simulink library "ddm"  (R2021b)
settings: Solver=VariableStepAuto  StartTime=0.0  StopTime=10.0  RelTol=1e-3
undefined symbols (not defined in the file): ADDM_FrTMTqDev_X_Nm, ADDM_RrTMTqDev_X_Nm, ENUM_ADASACCSTA_ERROR, ENUM_ADASACCSTA_OFF, ENUM_ADASACCSTA_STANDBY, ENUM_ALLOWMOV_ALLOWREADY, ENUM_APS, ENUM_BRKSTA_ERROR, ENUM_BRKSTA_OFF, ENUM_BRKSTA_ON, ENUM_BRKSW_INVALID, ENUM_BRKSW_OFF, ENUM_BRKSW_ON, ENUM_CHGPREACTERRSTA_OBCPRE, ENUM_DCDCFAULTSTA_ANYFAULTLV1, ENUM_DCDCFAULTSTA_ANYFAULTLV2, ENUM_DRIVETRAIN_AWD, ENUM_DRIVETRAIN_FWD, ENUM_DRIVETRAIN_RWD, ENUM_EDUDRTSTA_NORMAL, ENUM_EPBERROR_FAILED, ENUM_EPBSTA_APPLIED, ENUM_EPBSTA_RELEASED, ENUM_ESCAPSSta_APSUNAVAILABLE, ENUM_GEARACTUALPOSN_INVALID, ENUM_GEARACTUALPOSN_P, ENUM_HVBATTREADYPRE_READY, ENUM_HWRESETSTA_HWRESETING, ENUM_MCUWARN_LV0, ENUM_MCUWARN_LV1, ENUM_MCUWARN_LV2, ENUM_MCUWARN_LV3, ENUM_MCUWARN_NOERROR, ENUM_OBCFAULTSTA_ANYFAULT, ENUM_PAS_R2F2, ENUM_PDFAULT_BATTPDFAIL, ENUM_PDFAULT_DCDCDISABLE, ENUM_PDFAULT_MCUDISABLE, ENUM_PDFAULT_MCUDISCHRG, ENUM_POWERSTA_OFF, ENUM_POWERSTA_ON, ENUM_POWERSTA_READY, ENUM_POWERSTA_STANDBY, ENUM_PRESSINDI_LOW, ENUM_PUFAULT_BATTUPFAIL, ENUM_PUFAULT_DCDCENABLEFAIL, ENUM_PUFAULT_PRECHRGCHKFAIL, ENUM_PUFAULT_SAFETYCHKFAIL, ENUM_PWRSTASW_OFF, ENUM_PWRSTASW_OFFA, ENUM_PWRSTASW_OFFCHVCHRG, ENUM_PWRSTASW_OFFCLVCHRG, ENUM_PWRSTASW_ON, ENUM_PWRSTASW_ONHVCHRG, ENUM_PWRSTASW_READY, ENUM_PWRSTASW_STANDBY, ENUM_RAPSErrWarnSta_NORMAL, ENUM_RAPSErrWarnSta_RAPSERRLV1, ENUM_SHIFTCOMMAND_P, ENUM_SHIFTERERRSTA_PBUTTONFAILURE ... (+471)
libraries: hcu_lib x540, simulink x3
(part 3 of 26)

== system ddm/DDM/DDM_MCU_Signal_Selector ==
  BINP_CAN3_outputs : Inport  OutDataTypeStr=Bus: BINP_CAN3_outputs
  BINP_SYS_outputs : Inport  Port=2  OutDataTypeStr=Bus: BINP_SYS_outputs
  Bus Creator : BusCreator  Inputs=14
  Bus Selector : BusSelector  OutputSignals=VINP_CANMsgValidMCUBF1_flg,VINP_CANMsgValidMCUNF1_flg,VINP_MCUBF1RCErr_flg,VINP_MCUNF1RCErr_flg,VINP_MCUBF1CSErr_flg,VINP_MCUNF1CSErr_flg,VINP_CANMsgValidMCUBR1_flg,VINP_CANMsgValidMCUNR1_flg,VINP_MCUBR1RCErr_flg,VINP_MCUNR1RCErr_flg,VINP_MCUBR1CSErr_flg,VINP_MCUNR1CSErr_flg,VINP_MCUWarnFNidec_enum,VINP_MCUWarnRNidec_enum,VINP_MCUWarnF_enum,VINP_MCUWarnR_enum,VINP_FrMCUReady4Pre_flg,VINP_FrMCUReady4PreNidec_flg,VINP_RrMCUReady4Pre_flg,VINP_RrMCUReady4PreNidec_flg,VINP_FrMCUEnaSta_flg,VINP_FrMCUEnaStaNidec_flg,VINP_RrMCUEnaSta_flg,VINP_RrMCUEnaStaNidec_flg,VINP_FrMCUDCBusVolt_V,VINP_FrMCUDCBusVoltNidec_V,VINP_RrMCUDCBusVolt_V,VINP_RrMCUDCBusVoltNidec_V
  Bus Selector1 : BusSelector  OutputSignals=VINP_VehicleType_enum
  "DDM Signal Convert " : Subsystem  TreatAsAtomicUnit=on
  BDDM_CAN3MCU_outputs : Outport
  wires:
  BINP_CAN3_outputs/1 -> Bus Selector/1
  [VINP_MCUBF1RCErr_flg] -> "DDM Signal Convert "/3(VINP_MCUBF1RCErr_flg)
  [VINP_RrMCUDCBusVoltNidec_V] -> "DDM Signal Convert "/29(VINP_RrMCUDCBusVoltNidec_V)
  "DDM Signal Convert "/14(VDDM_RrMCUDCBusVolt_V) -> [VDDM_RrMCUDCBusVolt_V]
  [VINP_RrMCUReady4Pre_flg] -> "DDM Signal Convert "/20(VINP_RrMCUReady4Pre_flg)
  "DDM Signal Convert "/4(VDDM_CANMsgValidMCUR1_flg) -> [VDDM_CANMsgValidMCUR1_flg]
  "DDM Signal Convert "/6(VDDM_MCUR1CSErr_flg) -> [VDDM_MCUR1CSErr_flg]
  [VINP_MCUBF1CSErr_flg] -> "DDM Signal Convert "/5(VINP_MCUBF1CSErr_flg)
  [VINP_MCUBR1RCErr_flg] -> "DDM Signal Convert "/9(VINP_MCUBR1RCErr_flg)
  [VINP_MCUBR1CSErr_flg] -> "DDM Signal Convert "/11(VINP_MCUBR1CSErr_flg)
  [VINP_VehicleType_enum] -> "DDM Signal Convert "/13(VINP_VehicleType_enum)
  [VINP_RrMCUDCBusVolt_V] -> "DDM Signal Convert "/28(VINP_RrMCUDCBusVolt_V)
  [VINP_FrMCUEnaStaNidec_flg] -> "DDM Signal Convert "/23(VINP_FrMCUEnaStaNidec_flg)
  [VINP_MCUNR1RCErr_flg] -> "DDM Signal Convert "/10(VINP_MCUNR1RCErr_flg)
  "DDM Signal Convert "/7(VDDM_MCUWarnF_enum) -> [VDDM_MCUWarnF_enum]
  [VINP_MCUWarnR_enum] -> "DDM Signal Convert "/17(VINP_MCUWarnR_enum)
  [VINP_FrMCUReady4PreNidec_flg] -> "DDM Signal Convert "/19(VINP_FrMCUReady4PreNidec_flg)
  [VINP_MCUNR1CSErr_flg] -> "DDM Signal Convert "/12(VINP_MCUNR1CSErr_flg)
  [VINP_RrMCUEnaStaNidec_flg] -> "DDM Signal Convert "/25(VINP_RrMCUEnaStaNidec_flg)
  "DDM Signal Convert "/1(VDDM_CANMsgValidMCUF1_flg) -> [VDDM_CANMsgValidMCUF1_flg]
  [VINP_FrMCUReady4Pre_flg] -> "DDM Signal Convert "/18(VINP_FrMCUReady4Pre_flg)
  [VINP_MCUWarnRNidec_enum] -> "DDM Signal Convert "/15(VINP_MCUWarnRNidec_enum)
  "DDM Signal Convert "/13(VDDM_FrMCUDCBusVolt_V) -> [VDDM_FrMCUDCBusVolt_V]
  [VINP_CANMsgValidMCUNR1_flg] -> "DDM Signal Convert "/8(VINP_CANMsgValidMCUNR1_flg)
  [VINP_FrMCUDCBusVoltNidec_V] -> "DDM Signal Convert "/27(VINP_FrMCUDCBusVoltNidec_V)
  "DDM Signal Convert "/2(VDDM_MCUF1RCErr_flg) -> [VDDM_MCUF1RCErr_flg]
  [VINP_CANMsgValidMCUBR1_flg] -> "DDM Signal Convert "/7(VINP_CANMsgValidMCUBR1_flg)
  [VINP_CANMsgValidMCUNF1_flg] -> "DDM Signal Convert "/2(VINP_CANMsgValidMCUNF1_flg)
  [VINP_CANMsgValidMCUBF1_flg] -> "DDM Signal Convert "/1(VINP_CANMsgValidMCUBF1_flg)
  "DDM Signal Convert "/3(VDDM_MCUF1CSErr_flg) -> [VDDM_MCUF1CSErr_flg]
  [VINP_RrMCUEnaSta_flg] -> "DDM Signal Convert "/24(VINP_RrMCUEnaSta_flg)
  [VINP_MCUNF1RCErr_flg] -> "DDM Signal Convert "/4(VINP_MCUNF1RCErr_flg)
  "DDM Signal Convert "/10(VDDM_RrMCUReady4Pre_flg) -> [VDDM_RrMCUReady4Pre_flg]
  "DDM Signal Convert "/5(VDDM_MCUR1RCErr_flg) -> [VDDM_MCUR1RCErr_flg]
  "DDM Signal Convert "/12(VDDM_RrMCUEnaSta_flg) -> [VDDM_RrMCUEnaSta_flg]
  [VINP_MCUWarnF_enum] -> "DDM Signal Convert "/16(VINP_MCUWarnF_enum)
  "DDM Signal Convert "/9(VDDM_FrMCUReady4Pre_flg) -> [VDDM_FrMCUReady4Pre_flg]
  [VINP_MCUNF1CSErr_flg] -> "DDM Signal Convert "/6(VINP_MCUNF1CSErr_flg)
  "DDM Signal Convert "/8(VDDM_MCUWarnR_enum) -> [VDDM_MCUWarnR_enum]
  [VINP_FrMCUDCBusVolt_V] -> "DDM Signal Convert "/26(VINP_FrMCUDCBusVolt_V)
  [VINP_RrMCUReady4PreNidec_flg] -> "DDM Signal Convert "/21(VINP_RrMCUReady4PreNidec_flg)
  "DDM Signal Convert "/11(VDDM_FrMCUEnaSta_flg) -> [VDDM_FrMCUEnaSta_flg]
  [VINP_FrMCUEnaSta_flg] -> "DDM Signal Convert "/22(VINP_FrMCUEnaSta_flg)
  [VINP_MCUWarnFNidec_enum] -> "DDM Signal Convert "/14(VINP_MCUWarnFNidec_enum)
  Bus Selector/1 -> [VINP_CANMsgValidMCUBF1_flg]  "<VINP_CANMsgValidMCUBF1_flg>"
  Bus Selector/2 -> [VINP_CANMsgValidMCUNF1_flg]  "<VINP_CANMsgValidMCUNF1_flg>"
  Bus Selector/3 -> [VINP_MCUBF1RCErr_flg]  "<VINP_MCUBF1RCErr_flg>"
  Bus Selector/4 -> [VINP_MCUNF1RCErr_flg]  "<VINP_MCUNF1RCErr_flg>"
  Bus Selector/5 -> [VINP_MCUBF1CSErr_flg]  "<VINP_MCUBF1CSErr_flg>"
  Bus Selector/6 -> [VINP_MCUNF1CSErr_flg]  "<VINP_MCUNF1CSErr_flg>"
  Bus Selector/7 -> [VINP_CANMsgValidMCUBR1_flg]  "<VINP_CANMsgValidMCUBR1_flg>"
  Bus Selector/8 -> [VINP_CANMsgValidMCUNR1_flg]  "<VINP_CANMsgValidMCUNR1_flg>"
  Bus Selector/9 -> [VINP_MCUBR1RCErr_flg]  "<VINP_MCUBR1RCErr_flg>"
  Bus Selector/10 -> [VINP_MCUNR1RCErr_flg]  "<VINP_MCUNR1RCErr_flg>"
  Bus Selector/11 -> [VINP_MCUBR1CSErr_flg]  "<VINP_MCUBR1CSErr_flg>"
  Bus Selector/12 -> [VINP_MCUNR1CSErr_flg]  "<VINP_MCUNR1CSErr_flg>"
  Bus Selector/13 -> [VINP_MCUWarnFNidec_enum]  "<VINP_MCUWarnFNidec_enum>"
  Bus Selector/14 -> [VINP_MCUWarnRNidec_enum]  "<VINP_MCUWarnRNidec_enum>"
  Bus Selector/15 -> [VINP_MCUWarnF_enum]  "<VINP_MCUWarnF_enum>"
  Bus Selector/16 -> [VINP_MCUWarnR_enum]  "<VINP_MCUWarnR_enum>"
  Bus Selector/17 -> [VINP_FrMCUReady4Pre_flg]  "<VINP_FrMCUReady4Pre_flg>"
  Bus Selector/18 -> [VINP_FrMCUReady4PreNidec_flg]  "<VINP_FrMCUReady4PreNidec_flg>"
  Bus Selector/19 -> [VINP_RrMCUReady4Pre_flg]  "<VINP_RrMCUReady4Pre_flg>"
  Bus Selector/20 -> [VINP_RrMCUReady4PreNidec_flg]  "<VINP_RrMCUReady4PreNidec_flg>"
  Bus Selector/21 -> [VINP_FrMCUEnaSta_flg]  "<VINP_FrMCUEnaSta_flg>"
  Bus Selector/22 -> [VINP_FrMCUEnaStaNidec_flg]  "<VINP_FrMCUEnaStaNidec_flg>"
  Bus Selector/23 -> [VINP_RrMCUEnaSta_flg]  "<VINP_RrMCUEnaSta_flg>"
  Bus Selector/24 -> [VINP_RrMCUEnaStaNidec_flg]  "<VINP_RrMCUEnaStaNidec_flg>"
  Bus Selector/25 -> [VINP_FrMCUDCBusVolt_V]  "<VINP_FrMCUDCBusVolt_V>"
  Bus Selector/26 -> [VINP_FrMCUDCBusVoltNidec_V]  "<VINP_FrMCUDCBusVoltNidec_V>"
  Bus Selector/27 -> [VINP_RrMCUDCBusVolt_V]  "<VINP_RrMCUDCBusVolt_V>"
  Bus Selector/28 -> [VINP_RrMCUDCBusVoltNidec_V]  "<VINP_RrMCUDCBusVoltNidec_V>"
  BINP_SYS_outputs/1 -> Bus Selector1/1
  Bus Selector1/1 -> [VINP_VehicleType_enum]  "<VINP_VehicleType_enum>"
  Bus Creator/1 -> BDDM_CAN3MCU_outputs/1
  [VDDM_CANMsgValidMCUF1_flg] -> Bus Creator/1
  [VDDM_RrMCUDCBusVolt_V] -> Bus Creator/14
  [VDDM_FrMCUDCBusVolt_V] -> Bus Creator/13
  [VDDM_RrMCUEnaSta_flg] -> Bus Creator/12
  [VDDM_FrMCUEnaSta_flg] -> Bus Creator/11
  [VDDM_RrMCUReady4Pre_flg] -> Bus Creator/10
  [VDDM_FrMCUReady4Pre_flg] -> Bus Creator/9
  [VDDM_MCUWarnR_enum] -> Bus Creator/8
  [VDDM_MCUWarnF_enum] -> Bus Creator/7
  [VDDM_MCUR1CSErr_flg] -> Bus Creator/6
  [VDDM_MCUR1RCErr_flg] -> Bus Creator/5
  [VDDM_CANMsgValidMCUR1_flg] -> Bus Creator/4
  [VDDM_MCUF1CSErr_flg] -> Bus Creator/3
  [VDDM_MCUF1RCErr_flg] -> Bus Creator/2

== system ddm/DDM/DDM/APM ==
  VAPM_USSStaFCL_flg : Inport
  VAPM_USSStaFML_flg : Inport  Port=2
  VAPM_USSStaFMR_flg : Inport  Port=3
  VAPM_USSStaFCR_flg : Inport  Port=4
  VAPM_USSStaRCL_flg : Inport  Port=5
  VAPM_USSStaRML_flg : Inport  Port=6
  VAPM_USSStaRMR_flg : Inport  Port=7
  VAPM_USSStaRCR_flg : Inport  Port=8
  VAPM_USSStaFLL_flg : Inport  Port=9
  VAPM_USSStaFLR_flg : Inport  Port=10
  VAPM_USSStaRLL_flg : Inport  Port=11
  VAPM_USSStaRLR_flg : Inport  Port=12
  DTC_clear_request : Inport  Port=13
  VPMM_SysPwrSta_enum : Inport  Port=14
  VAPM_SNSRLayout_enum : Inport  Port=15
  DTC_Info{,1..11} (12 alike) : hcu_lib/Basic_Blocks/DTC_Info
  Ground{,1..11} (12 alike) : Ground
  Subsystem : Subsystem
  Subsystem1 : Subsystem
  Subsystem10 : Subsystem
  Subsystem11 : Subsystem
  Subsystem2 : Subsystem
  Subsystem3 : Subsystem
  Subsystem4 : Subsystem
  Subsystem5 : Subsystem
  Subsystem6 : Subsystem
  Subsystem7 : Subsystem
  Subsystem8 : Subsystem
  Subsystem9 : Subsystem
  VDDM_FCLUSSDTC_raw32 : Outport
  VDDM_FMLUSSDTC_raw32 : Outport  Port=2
  VDDM_FMRUSSDTC_raw32 : Outport  Port=3
  VDDM_FCRUSSDTC_raw32 : Outport  Port=4
  VDDM_RCLUSSDTC_raw32 : Outport  Port=5
  VDDM_RMLUSSDTC_raw32 : Outport  Port=6
  VDDM_RMRUSSDTC_raw32 : Outport  Port=7
  VDDM_RCRUSSDTC_raw32 : Outport  Port=8
  VDDM_FLLUSSDTC_raw32 : Outport  Port=9
  VDDM_FLRUSSDTC_raw32 : Outport  Port=10
  VDDM_RLLUSSDTC_raw32 : Outport  Port=11
  VDDM_RLRUSSDTC_raw32 : Outport  Port=12
  wires:
  [VAPM_SNSRLayout_enum] -> Subsystem11/3(VAPM_SNSRLayout_enum)
  [DTC_clear_request] -> DTC_Info11/4
  Subsystem11/2(CFS_flg) -> DTC_Info11/3
  Subsystem11/1(Pass_flg) -> DTC_Info11/2
  [VAPM_SNSRLayout_enum] -> Subsystem10/3(VAPM_SNSRLayout_enum)
  [DTC_clear_request] -> DTC_Info10/4
  Subsystem10/2(CFS_flg) -> DTC_Info10/3
  Subsystem10/1(Pass_flg) -> DTC_Info10/2
  [VAPM_SNSRLayout_enum] -> Subsystem9/3(VAPM_SNSRLayout_enum)
  [DTC_clear_request] -> DTC_Info9/4
  Subsystem9/2(CFS_flg) -> DTC_Info9/3
  Subsystem9/1(Pass_flg) -> DTC_Info9/2
  Ground9/1 -> DTC_Info9/1
  [VAPM_SNSRLayout_enum] -> Subsystem8/3(VAPM_SNSRLayout_enum)
  [DTC_clear_request] -> DTC_Info8/4
  Subsystem8/2(CFS_flg) -> DTC_Info8/3
  Subsystem8/1(Pass_flg) -> DTC_Info8/2
  [VAPM_SNSRLayout_enum] -> Subsystem7/3(VAPM_SNSRLayout_enum)
  [DTC_clear_request] -> DTC_Info7/4
  Subsystem7/2(CFS_flg) -> DTC_Info7/3
  Subsystem7/1(Pass_flg) -> DTC_Info7/2
  [VAPM_SNSRLayout_enum] -> Subsystem6/3(VAPM_SNSRLayout_enum)
  [DTC_clear_request] -> DTC_Info6/4
  Subsystem6/2(CFS_flg) -> DTC_Info6/3
  Subsystem6/1(Pass_flg) -> DTC_Info6/2
  [VAPM_SNSRLayout_enum] -> Subsystem5/3(VAPM_SNSRLayout_enum)
  [DTC_clear_request] -> DTC_Info5/4
  Subsystem5/2(CFS_flg) -> DTC_Info5/3
  Subsystem5/1(Pass_flg) -> DTC_Info5/2
  [VAPM_SNSRLayout_enum] -> Subsystem4/3(VAPM_SNSRLayout_enum)
  [DTC_clear_request] -> DTC_Info4/4
  Subsystem4/2(CFS_flg) -> DTC_Info4/3
  Subsystem4/1(Pass_flg) -> DTC_Info4/2
  Ground4/1 -> DTC_Info4/1
  [VAPM_SNSRLayout_enum] -> Subsystem3/3(VAPM_SNSRLayout_enum)
  [DTC_clear_request] -> DTC_Info3/4
  Subsystem3/2(CFS_flg) -> DTC_Info3/3
  Subsystem3/1(Pass_flg) -> DTC_Info3/2
  [VAPM_SNSRLayout_enum] -> Subsystem2/3(VAPM_SNSRLayout_enum)
  [DTC_clear_request] -> DTC_Info2/4
  [VPMM_SysPwrSta_enum] -> Subsystem2/2(VPMM_SysPwrSta_enum)
  VAPM_USSStaFMR_flg/1 -> Subsystem2/1(USSSta_flg)
  Subsystem2/2(CFS_flg) -> DTC_Info2/3
  Subsystem2/1(Pass_flg) -> DTC_Info2/2
  [VAPM_SNSRLayout_enum] -> Subsystem1/3(VAPM_SNSRLayout_enum)
  [VAPM_SNSRLayout_enum] -> Subsystem/3(VAPM_SNSRLayout_enum)
  VAPM_SNSRLayout_enum/1 -> [VAPM_SNSRLayout_enum]
  DTC_Info/1 -> VDDM_FCLUSSDTC_raw32/1  "VDDM_FCLUSSDTC_raw32"
  Ground/1 -> DTC_Info/1
  DTC_clear_request/1 -> [DTC_clear_request]
  [DTC_clear_request] -> DTC_Info/4
  [DTC_clear_request] -> DTC_Info1/4
  VAPM_USSStaFML_flg/1 -> Subsystem1/1(USSSta_flg)
  Ground1/1 -> DTC_Info1/1
  DTC_Info1/1 -> VDDM_FMLUSSDTC_raw32/1  "VDDM_FMLUSSDTC_raw32"
  DTC_Info2/1 -> VDDM_FMRUSSDTC_raw32/1  "VDDM_FMRUSSDTC_raw32"
  Ground2/1 -> DTC_Info2/1
  Ground3/1 -> DTC_Info3/1
  DTC_Info3/1 -> VDDM_FCRUSSDTC_raw32/1  "VDDM_FCRUSSDTC_raw32"
  DTC_Info4/1 -> VDDM_RCLUSSDTC_raw32/1  "VDDM_RCLUSSDTC_raw32"
  Ground5/1 -> DTC_Info5/1
  DTC_Info5/1 -> VDDM_RMLUSSDTC_raw32/1  "VDDM_RMLUSSDTC_raw32"
  DTC_Info6/1 -> VDDM_RMRUSSDTC_raw32/1  "VDDM_RMRUSSDTC_raw32"
  Ground6/1 -> DTC_Info6/1
  Ground7/1 -> DTC_Info7/1
  DTC_Info7/1 -> VDDM_RCRUSSDTC_raw32/1  "VDDM_RCRUSSDTC_raw32"
  DTC_Info8/1 -> VDDM_FLLUSSDTC_raw32/1  "VDDM_FLLUSSDTC_raw32"
  Ground8/1 -> DTC_Info8/1
  DTC_Info9/1 -> VDDM_FLRUSSDTC_raw32/1  "VDDM_FLRUSSDTC_raw32"
  DTC_Info10/1 -> VDDM_RLLUSSDTC_raw32/1  "VDDM_RLLUSSDTC_raw32"
  Ground10/1 -> DTC_Info10/1
  Ground11/1 -> DTC_Info11/1
  DTC_Info11/1 -> VDDM_RLRUSSDTC_raw32/1  "VDDM_RLRUSSDTC_raw32"
  VAPM_USSStaFCL_flg/1 -> Subsystem/1(USSSta_flg)
  Subsystem/1(Pass_flg) -> DTC_Info/2
  Subsystem/2(CFS_flg) -> DTC_Info/3
  Subsystem1/1(Pass_flg) -> DTC_Info1/2
  Subsystem1/2(CFS_flg) -> DTC_Info1/3
  [VPMM_SysPwrSta_enum] -> Subsystem/2(VPMM_SysPwrSta_enum)
  VPMM_SysPwrSta_enum/1 -> [VPMM_SysPwrSta_enum]
  [VPMM_SysPwrSta_enum] -> Subsystem1/2(VPMM_SysPwrSta_enum)
  [VPMM_SysPwrSta_enum] -> Subsystem3/2(VPMM_SysPwrSta_enum)
  VAPM_USSStaFCR_flg/1 -> Subsystem3/1(USSSta_flg)
  [VPMM_SysPwrSta_enum] -> Subsystem4/2(VPMM_SysPwrSta_enum)
  VAPM_USSStaRCL_flg/1 -> Subsystem4/1(USSSta_flg)
  [VPMM_SysPwrSta_enum] -> Subsystem5/2(VPMM_SysPwrSta_enum)
  VAPM_USSStaRML_flg/1 -> Subsystem5/1(USSSta_flg)
  [VPMM_SysPwrSta_enum] -> Subsystem6/2(VPMM_SysPwrSta_enum)
  VAPM_USSStaRMR_flg/1 -> Subsystem6/1(USSSta_flg)
  [VPMM_SysPwrSta_enum] -> Subsystem7/2(VPMM_SysPwrSta_enum)
  VAPM_USSStaRCR_flg/1 -> Subsystem7/1(USSSta_flg)
  [VPMM_SysPwrSta_enum] -> Subsystem8/2(VPMM_SysPwrSta_enum)
  VAPM_USSStaFLL_flg/1 -> Subsystem8/1(USSSta_flg)
  [VPMM_SysPwrSta_enum] -> Subsystem9/2(VPMM_SysPwrSta_enum)
  VAPM_USSStaFLR_flg/1 -> Subsystem9/1(USSSta_flg)
  [VPMM_SysPwrSta_enum] -> Subsystem10/2(VPMM_SysPwrSta_enum)
  VAPM_USSStaRLL_flg/1 -> Subsystem10/1(USSSta_flg)
  [VPMM_SysPwrSta_enum] -> Subsystem11/2(VPMM_SysPwrSta_enum)
  VAPM_USSStaRLR_flg/1 -> Subsystem11/1(USSSta_flg)

== system ddm/DDM/DDM/BCM ==
  VBCM_DiagHCrash_flg : Inport
  VBCM_DiagFLTS_flg : Inport  Port=2
  VBCM_DiagFRTS_flg : Inport  Port=3
  VBCM_DiagRLTS_flg : Inport  Port=4
  VBCM_DiagRRTS_flg : Inport  Port=5
  DTC_clear_request : Inport  Port=6
  DTC_Info{,1..4} (5 alike) : hcu_lib/Basic_Blocks/DTC_Info
  Ground{,1..4} (5 alike) : Ground
  Logical Operator{1..5} (5 alike) : Logic  Operator=NOT  AllPortsSameDT=off  OutDataTypeStr=boolean
  VDDM_DiagHCrashDTC_raw32 : Outport
  VDDM_DiagFLTSDTC_raw32 : Outport  Port=2
  VDDM_DiagFRTSDTC_raw32 : Outport  Port=3
  VDDM_DiagRLTSDTC_raw32 : Outport  Port=4
  VDDM_DiagRRTSDTC_raw32 : Outport  Port=5
  wires:
  [DTC_clear_request] -> DTC_Info/4
  [DTC_clear_request] -> DTC_Info1/4
  [DTC_clear_request] -> DTC_Info4/4
  [DTC_clear_request] -> DTC_Info3/4
  [DTC_clear_request] -> DTC_Info2/4
  DTC_clear_request/1 -> [DTC_clear_request]
  VBCM_DiagRRTS_flg/1 -> Logical Operator5/1, DTC_Info4/3
  Ground4/1 -> DTC_Info4/1
  Logical Operator5/1 -> DTC_Info4/2
  DTC_Info4/1 -> VDDM_DiagRRTSDTC_raw32/1  "VDDM_DiagRRTSDTC_raw32"
  DTC_Info3/1 -> VDDM_DiagRLTSDTC_raw32/1  "VDDM_DiagRLTSDTC_raw32"
  Logical Operator4/1 -> DTC_Info3/2
  Ground3/1 -> DTC_Info3/1
  VBCM_DiagRLTS_flg/1 -> DTC_Info3/3, Logical Operator4/1
  VBCM_DiagFRTS_flg/1 -> Logical Operator3/1, DTC_Info2/3
  Ground2/1 -> DTC_Info2/1
  Logical Operator3/1 -> DTC_Info2/2
  DTC_Info2/1 -> VDDM_DiagFRTSDTC_raw32/1  "VDDM_DiagFRTSDTC_raw32"
  DTC_Info1/1 -> VDDM_DiagFLTSDTC_raw32/1  "VDDM_DiagFLTSDTC_raw32"
  Logical Operator2/1 -> DTC_Info1/2
  Ground1/1 -> DTC_Info1/1
  VBCM_DiagFLTS_flg/1 -> DTC_Info1/3, Logical Operator2/1
  Logical Operator1/1 -> DTC_Info/2
  VBCM_DiagHCrash_flg/1 -> DTC_Info/3, Logical Operator1/1
  Ground/1 -> DTC_Info/1
  DTC_Info/1 -> VDDM_DiagHCrashDTC_raw32/1  "VDDM_DiagHCrashDTC_raw32"
